simulink model "WDGTTCCalculation"  (R2024a)
settings: configuration reference "csMultiInstance" (kept outside this file)
undefined symbols (not defined in the file or in its folder): Distance_Max, Distance_Min, headwayOffset, Ts, TTC_Max, TTC_Min, Velocity_Max, Velocity_Min
Description:
  | Software unit to calculate TTC
settings Model: DataDictionary=DD_WDGTTCCalculation.sldd  EnableAccessToBaseWorkspace=off  Creator=The MathWorks, Inc.  LastModifiedBy=The MathWorks, Inc.
settings ConfigSetRef: SourceName=csMultiInstance

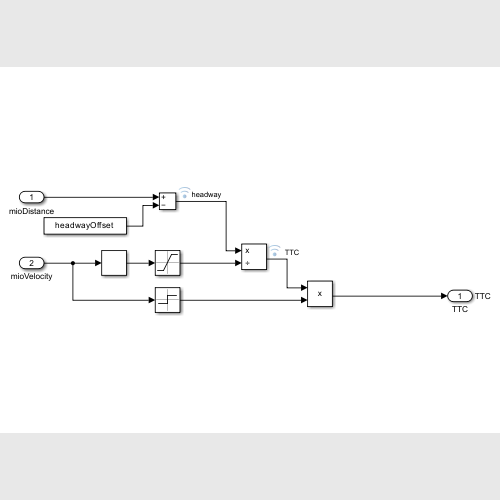
[thumbnail: Simulink's stored preview of the top-level diagram]
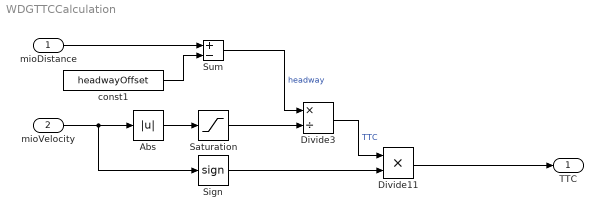
== system WDGTTCCalculation ==
  mioDistance : Inport  OutMin=Distance_Min  OutMax=Distance_Max  OutDataTypeStr=Distance_DType  Unit=m  PortDimensions=Distance_Dimensions  SampleTime=Ts
  mioVelocity : Inport  Port=2  OutMin=Velocity_Min  OutMax=Velocity_Max  OutDataTypeStr=Velocity_DType  Unit=m/s  PortDimensions=Velocity_Dimensions  SampleTime=Ts
  Abs : Abs  SaturateOnIntegerOverflow=off
  Divide11 : Product  Inputs=**
  Divide3 : Product  Inputs=*/
  Saturation : Saturate  UpperLimit=100  LowerLimit=0.01
  Sign : Signum
  Sum : Sum  Inputs=+-
  const1 : Constant  Value=headwayOffset  SampleTime=-1
  TTC : Outport  SignalName=TTC  OutMin=TTC_Min  OutMax=TTC_Max  OutDataTypeStr=TTC_DType  Unit=s  PortDimensions=TTC_Dimensions  SampleTime=Ts  VectorParamsAs1DForOutWhenUnconnected=off
  wires:
  Divide11/1 -> TTC/1
  Saturation/1 -> Divide3/2
  mioDistance/1 -> Sum/1
  Sign/1 -> Divide11/2
  mioVelocity/1 -> Abs/1, Sign/1
  Sum/1 -> Divide3/1  "headway"
  Abs/1 -> Saturation/1
  Divide3/1 -> Divide11/1  "TTC"
  const1/1 -> Sum/2
